simulink model "lindiscrmodel_lqr_uu_report"  (R2019a)
settings: Solver=VariableStepAuto  StartTime=0.0  StopTime=15  RelTol=1e-3
InitFcn:
  | lindiscrmodel
values from neighbouring files (symbols this model uses):
  Ts = 0.01    [lindiscrmodel.m]
undefined symbols (not defined in the file or in its folder): Discrete, K2, linmat, R_kal, Time
libraries: ctrlSharedLib x1
settings Model: Creator=jessi  LastModifiedBy=jessi

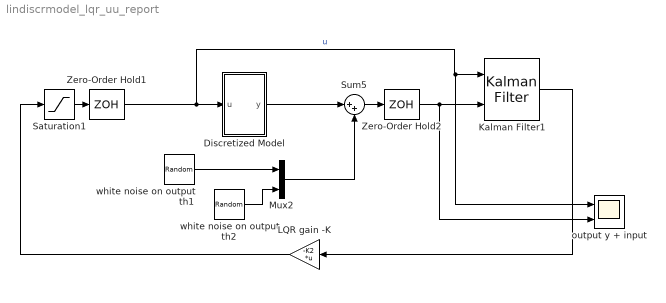
== system lindiscrmodel_lqr_uu_report ==
  Discretized Model : Subsystem
  Kalman Filter1 : ctrlSharedLib/Kalman Filter  TimeDomain=Discrete-Time  UseCurrentEstimator=on  ModelSource=Individual A, B, C, D matrices  ModelSourceVariable=sysd2  A=linmat.A2  B=linmat.B2  C=linmat.C2  D=linmat.D2  NumberOfStates=1  NumberOfInputs=1  NumberOfOutputs=1  InitialEstimateSource=Dialog  X0=[0;0.05;0;0]  P0=10  UseK=off  UseGH=off  NumberOfProcessNoiseInputs=1  G=1  TimeInvariantG=on  H=0  TimeInvariantH=on  Q=0.000001*diag([1 1 1 1])  TimeInvariantQ=on  R=R_kal  TimeInvariantR=on  N=0  TimeInvariantN=on  AddInputPort=on  AddEnablePort=off  OutputEstimatedY=off  OutputP=off  Ts=Ts
      settings: SourceProductBaseCode=CT
  LQR gain -K : Gain  Gain=-K2  Multiplication=Matrix(K*u)
  Mux2 : Mux  Inputs=2
  Saturation1 : Saturate  UpperLimit=1  LowerLimit=-1
  Sum5 : Sum  Inputs=|++
  Zero-Order Hold1 : ZeroOrderHold  SampleTime=Ts
  Zero-Order Hold2 : ZeroOrderHold  SampleTime=Ts
  output y + input : Scope  NumInputPorts=2
  white noise on output th1 : RandomNumber  Variance=1e-7  SampleTime=0.01
  white noise on output th2 : RandomNumber  Variance=1e-7  SampleTime=0.01
  wires:
  white noise on output th1/1 -> Mux2/1
  white noise on output th2/1 -> Mux2/2
  Mux2/1 -> Sum5/2
  Sum5/1 -> Zero-Order Hold2/1
  Saturation1/1 -> Zero-Order Hold1/1
  Discretized Model/1(y) -> Sum5/1
  Kalman Filter1/1 -> LQR gain -K/1
  Zero-Order Hold1/1 -> output y + input/1, Kalman Filter1/1, Discretized Model/1(u)  "u"
  Zero-Order Hold2/1 -> output y + input/2, Kalman Filter1/2
  LQR gain -K/1 -> Saturation1/1

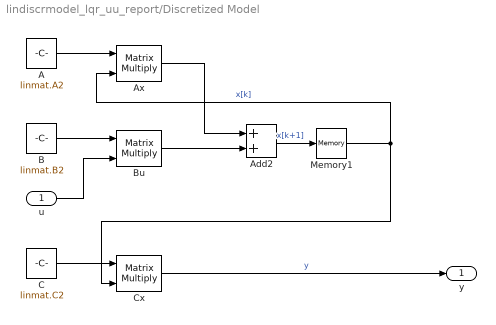
== system lindiscrmodel_lqr_uu_report/Discretized Model ==
  u : Inport
  A : Constant  Value=linmat.A2  SampleTime=Ts
  Add2 : Sum
  Ax : Product  Multiplication=Matrix(*)
  B : Constant  Value=linmat.B2  SampleTime=Ts
  Bu : Product  Multiplication=Matrix(*)
  C : Constant  Value=linmat.C2  SampleTime=Ts
  Cx : Product  Multiplication=Matrix(*)
  Memory1 : Memory  InitialCondition=[0;0.05;0;0]
  y : Outport
  wires:
  B/1 -> Bu/1
  Memory1/1 -> Cx/2, Ax/2  "x[k]"
  Add2/1 -> Memory1/1  "x[k+1]"
  C/1 -> Cx/1
  A/1 -> Ax/1
  u/1 -> Bu/2
  Ax/1 -> Add2/1
  Bu/1 -> Add2/2
  Cx/1 -> y/1  "y"
